simulink model "SimulacionMOAConLaplace"  (R2022a)
settings: Solver=VariableStepAuto  StartTime=0.0  StopTime=10  RelTol=1e-3
settings Model: Creator=Asus-PC  LastModifiedBy=Asus-PC

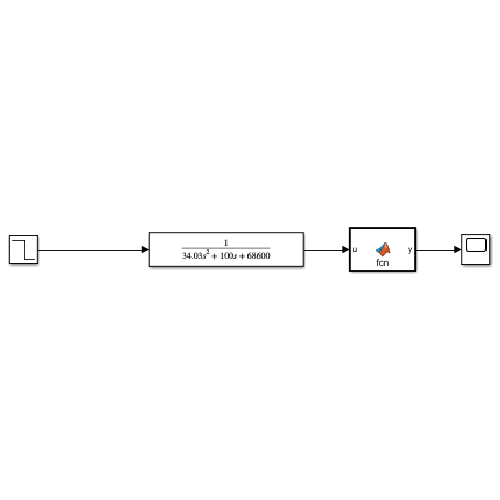
[thumbnail: Simulink's stored preview of the top-level diagram]
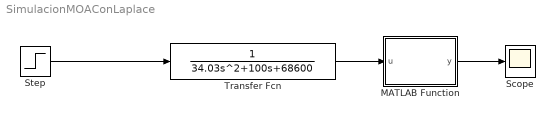
== system SimulacionMOAConLaplace ==
  MATLAB Function : MATLAB Function  TreatAsAtomicUnit=on
  Scope : Scope
  Step : Step  Time=0.01  Before=4080  After=0  SampleTime=0
  Transfer Fcn : TransferFcn  Denominator=[34.03 100 68600]
  wires:
  Step/1 -> Transfer Fcn/1
  Transfer Fcn/1 -> MATLAB Function/1(u)
  MATLAB Function/1(y) -> Scope/1

== matlab function SimulacionMOAConLaplace/MATLAB Function ==
  data: u input; y output
function y = fcn(u)
y = u;
fprintf('\n %f',y);
